simulink model "HARV2"  (Simulink 9.3)
settings: Solver=VariableStepAuto  StartTime=0.0  StopTime=1000  FixedStep=0.01  MaxStep=0.01  MinStep=0.000001  RelTol=1e-3
undefined symbols (not defined in the file or in its folder): ad, ae, airlib, b, B747, cbar, DT, eqm, fms, GM, gr, hlp, m, S
libraries: simulink x1
(part 2 of 2)

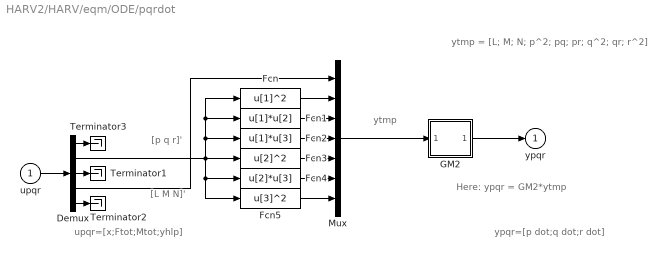
== system HARV2/HARV/eqm/ODE/pqrdot ==
  note: [p q r]'
  note: [L M N]'
  note: Here: ypqr = GM2*ytmp
  note: ytmp
  note: ypqr=[p dot;q dot;r dot]
  note: upqr=[x;Ftot;Mtot;yhlp]
  note: ytmp = [L; M; N; p^2; pq; pr; q^2; qr; r^2]
  upqr : Inport
  Demux : Demux  Outputs=[3 3 9 3 11]
  Fcn : Fcn  Expr=u[1]^2
  Fcn1 : Fcn  Expr=u[1]*u[2]
  Fcn2 : Fcn  Expr=u[1]*u[3]
  Fcn3 : Fcn  Expr=u[2]^2
  Fcn4 : Fcn  Expr=u[2]*u[3]
  Fcn5 : Fcn  Expr=u[3]^2
  "GM2 " : Subsystem  mask(State Space){M=GM}
      mask prompts: M "Matrix"
      mask Display: disp('Matrix\nGain')
  Mux : Mux  Inputs=[3 1 1 1 1 1 1]
  Terminator1 : Terminator
  Terminator2 : Terminator
  Terminator3 : Terminator
  ypqr : Outport
  wires:
  upqr/1 -> Demux/1
  Demux/1 -> Terminator3/1
  Demux/5 -> Terminator2/1
  Demux/3 -> Terminator1/1
  Demux/2 -> Fcn1/1, Fcn/1, Fcn2/1, Fcn4/1, Fcn5/1, Fcn3/1
  Demux/4 -> Mux/1
  Fcn/1 -> Mux/2
  Fcn1/1 -> Mux/3
  Fcn2/1 -> Mux/4
  Fcn3/1 -> Mux/5
  Fcn4/1 -> Mux/6
  Fcn5/1 -> Mux/7
  "GM2 "/1(Out1) -> ypqr/1
  Mux/1 -> "GM2 "/1(In1)

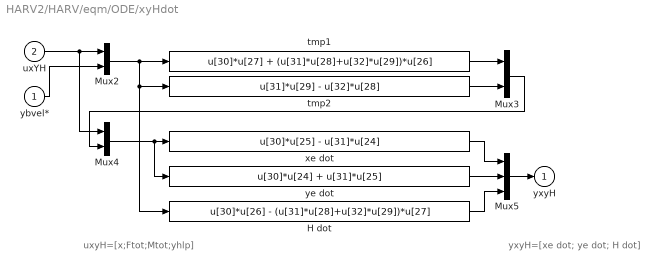
== system HARV2/HARV/eqm/ODE/xyHdot ==
  note: yxyH=[xe dot; ye dot; H dot]
  note: uxyH=[x;Ftot;Mtot;yhlp]
  ybvel* : Inport
  uxYH : Inport  Port=2
  H dot : Fcn  Expr=u[30]*u[26] - (u[31]*u[28]+u[32]*u[29])*u[27]
  Mux2 : Mux  Inputs=[29 3]
  Mux3 : Mux  Inputs=2
  Mux4 : Mux  Inputs=[29 2]
  Mux5 : Mux  Inputs=3
  tmp1 : Fcn  Expr=u[30]*u[27] + (u[31]*u[28]+u[32]*u[29])*u[26]
  tmp2 : Fcn  Expr=u[31]*u[29] - u[32]*u[28]
  xe dot : Fcn  Expr=u[30]*u[25] - u[31]*u[24]
  ye dot : Fcn  Expr=u[30]*u[24] + u[31]*u[25]
  yxyH : Outport
  wires:
  tmp1/1 -> Mux3/1
  H dot/1 -> Mux5/3
  xe dot/1 -> Mux5/1
  tmp2/1 -> Mux3/2
  ye dot/1 -> Mux5/2
  Mux5/1 -> yxyH/1
  Mux4/1 -> ye dot/1, xe dot/1
  Mux2/1 -> H dot/1, tmp2/1, tmp1/1
  Mux3/1 -> Mux4/2
  ybvel*/1 -> Mux2/2
  uxYH/1 -> Mux4/1, Mux2/1

== system HARV2/HARV/eqm/ODE/pqrdot/GM2  ==
  In1 : Inport
  Matrix Gain : StateSpace  A=[]  B=[]  C=[]  D=GM  InitialCondition=0
  Out1 : Outport
  wires:
  Matrix Gain/1 -> Out1/1
  In1/1 -> Matrix Gain/1
